simulink model "motor"  (R2016b)
settings: Solver=VariableStepAuto  StartTime=0.0  StopTime=10.0  RelTol=1e-3
settings Model: Creator=lqy  LastModifiedBy=lqy

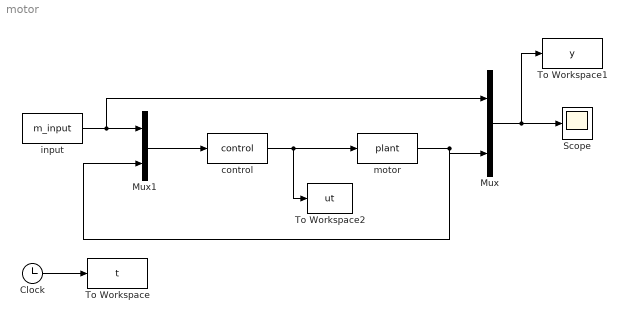
== system motor ==
  Clock : Clock
  Mux : Mux  Inputs=2
  Mux1 : Mux  Inputs=2
  Scope : Scope
  To Workspace : ToWorkspace  VariableName=t  SampleTime=-1
  To Workspace1 : ToWorkspace  VariableName=y  SampleTime=-1
  To Workspace2 : ToWorkspace  VariableName=ut  SampleTime=-1
  control : S-Function  FunctionName=control  SFunctionDeploymentMode=off  EnableBusSupport=off
  input : S-Function  FunctionName=m_input  SFunctionDeploymentMode=off  EnableBusSupport=off
  motor : S-Function  FunctionName=plant  SFunctionDeploymentMode=off  EnableBusSupport=off
  wires:
  control/1 -> To Workspace2/1, motor/1
  input/1 -> Mux/1, Mux1/1
  Mux1/1 -> control/1
  motor/1 -> Mux/2, Mux1/2
  Mux/1 -> To Workspace1/1, Scope/1
  Clock/1 -> To Workspace/1
